simulink model "Aufgabe2_2"  (R2020a)
settings: Solver=ode45  StartTime=0.0  StopTime=10  FixedStep=1e-5  RelTol=1e-9
undefined symbols (not defined in the file or in its folder): A0, a0, A1, B0, b0, B1, bf, bp, Fe
settings Model: Creator=Ravi Plenzdorf  LastModifiedBy=seife
settings DataIOCC: ReturnWorkspaceOutputs=off

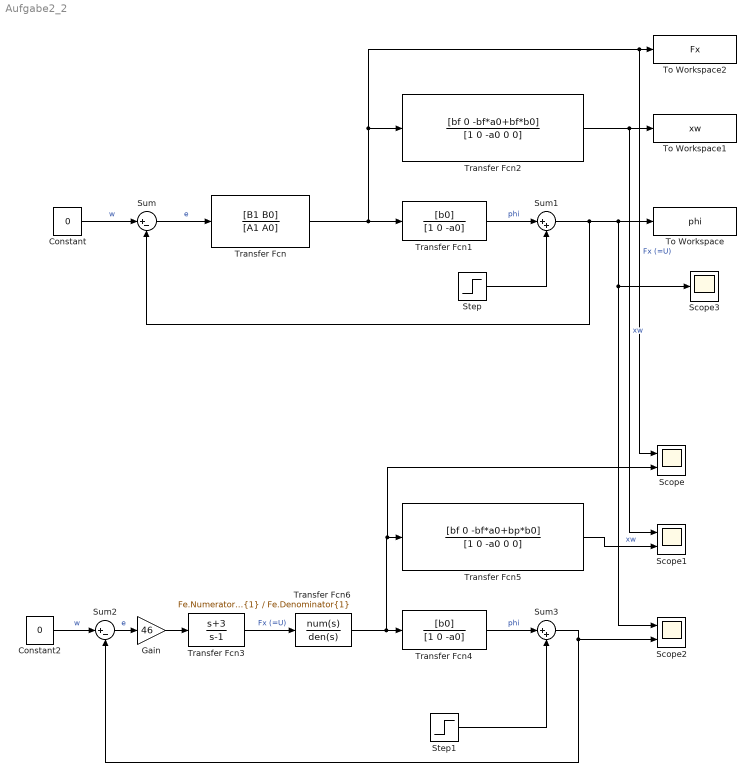
== system Aufgabe2_2 ==
  Constant : Constant  Value=0
  Constant2 : Constant  Value=0
  Gain : Gain  Gain=46
  Scope : Scope  NumInputPorts=2
  Scope1 : Scope  NumInputPorts=2
  Scope2 : Scope  NumInputPorts=2
  Scope3 : Scope
  Step : Step  After=0.017  SampleTime=0
  Step1 : Step  After=0.017  SampleTime=0
  Sum : Sum  Inputs=|+-
  Sum1 : Sum  Inputs=|++
  Sum2 : Sum  Inputs=|+-
  Sum3 : Sum  Inputs=|++
  To Workspace : ToWorkspace  VariableName=phi  SaveFormat=Timeseries  SampleTime=-1
  To Workspace1 : ToWorkspace  VariableName=xw  SaveFormat=Timeseries  SampleTime=-1
  To Workspace2 : ToWorkspace  VariableName=Fx  SaveFormat=Timeseries  SampleTime=-1
  Transfer Fcn : TransferFcn  Numerator=[B1 B0]  Denominator=[A1 A0]
  Transfer Fcn1 : TransferFcn  Numerator=[b0]  Denominator=[1 0 -a0]
  Transfer Fcn2 : TransferFcn  Numerator=[bf 0 -bf*a0+bf*b0]  Denominator=[1 0 -a0 0 0]
  Transfer Fcn3 : TransferFcn  Numerator=[1 3]  Denominator=[1 -1]
  Transfer Fcn4 : TransferFcn  Numerator=[b0]  Denominator=[1 0 -a0]
  Transfer Fcn5 : TransferFcn  Numerator=[bf 0 -bf*a0+bp*b0]  Denominator=[1 0 -a0 0 0]
  Transfer Fcn6 : TransferFcn  Numerator=Fe.Numerator{1}  Denominator=Fe.Denominator{1}
  wires:
  Constant/1 -> Sum/1  "w"
  Sum/1 -> Transfer Fcn/1  "e"
  Transfer Fcn2/1 -> To Workspace1/1, Scope1/1  "xw"
  Transfer Fcn1/1 -> Sum1/1  "phi"
  Sum1/1 -> To Workspace/1, Scope3/1, Scope2/1, Sum/2
  Transfer Fcn5/1 -> Scope1/2  "xw"
  Transfer Fcn4/1 -> Sum3/1  "phi"
  Sum3/1 -> Scope2/2, Sum2/2
  Gain/1 -> Transfer Fcn3/1
  Constant2/1 -> Sum2/1  "w"
  Transfer Fcn3/1 -> Transfer Fcn6/1  "Fx (=U)"
  Sum2/1 -> Gain/1  "e"
  Step1/1 -> Sum3/2
  Transfer Fcn/1 -> Scope/1, To Workspace2/1, Transfer Fcn2/1, Transfer Fcn1/1  "Fx (=U)"
  Step/1 -> Sum1/2
  Transfer Fcn6/1 -> Scope/2, Transfer Fcn5/1, Transfer Fcn4/1
